simulink model "PID_GM_LastStoer_Kaskadenregler"  (R2021a)
settings: Solver=ode45  StartTime=0.0  StopTime=0.500  RelTol=1e-3  EnableMultiTasking=on
libraries: Regler x3
settings Model: Creator=zimmerma  LastModifiedBy=Manoli
settings SolverCC: AlgebraicLoopSolver=TrustRegion
settings DataIOCC: LimitDataPoints=on  SaveFormat=Array  SignalLoggingSaveFormat=ModelDataLogs  ReturnWorkspaceOutputs=off
settings OptimizationCC: ExpressionDepthLimit=2147483647  InitFltsAndDblsToZero=on  LifeSpan=inf
settings DebuggingCC: SaveWithParameterizedLinksMsg=none  UnderspecifiedInitializationDetection=Classic  MergeDetectMultiDrivingBlocksExec=none  SignalResolutionControl=TryResolveAllWithWarning  MultiTaskDSMMsg=warning  MultiTaskCondExecSysMsg=none  AllowSymbolicDim=off  StateNameClashWarn=warning  SFUnexpectedBacktrackingDiag=warning  SFNoUnconditionalDefaultTransitionDiag=warning  SFExecutionAtInitializationDiag=none  SFMachineParentedDataDiag=warning  ArithmeticOperatorsInVariantConditions=warning
settings HardwareCC: ProdBitPerPointer=32  ProdBitPerSizeT=32  ProdBitPerPtrDiffT=32  ProdLargestAtomicFloat=None  ProdIntDivRoundTo=Undefined  ProdEndianess=Unspecified  ProdWordSize=32  ProdHWDeviceType=32-bit Generic  TargetUnknown=on
settings ModelReferenceCC: PropagateSignalLabelsOutOfModel=off
settings SFSimCC: SimUseLocalCustomCode=off  CustomCodeUndefinedFunction=UseInterfaceOnly
settings RTWCC: RTWUseLocalCustomCode=off
settings CodeAppCC: StateflowObjectComments=on
settings GRTTargetCC: TargetFcnLib=ansi_tfl_tmw.mat  TargetLangStandard=C89/C90 (ANSI)  CombineOutputUpdateFcns=off  GRTInterface=on
settings ConfigComp: CovMetricSettings=dw  CovSaveCumulativeToWorkspaceVar=on  CovSaveSingleToWorkspaceVar=on  CovExternalEMLEnable=off

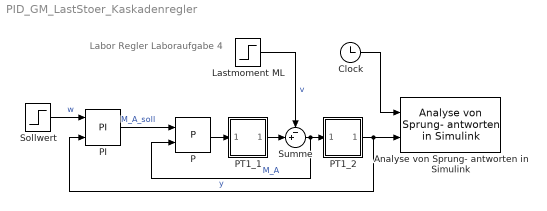
== system PID_GM_LastStoer_Kaskadenregler ==
  note: Labor Regler
      | Laboraufgabe 4
  Analyse von Sprung- antworten in Simulink : Regler/Analyse von Sprung- antworten in Simulink  tol=5
  Clock : Clock
  Lastmoment ML : Step  Time=0.200  SampleTime=0
  P : Regler/P  kp=1
  PI : Regler/PI  kp=10  Tn=100 / 1000
  PT1_1 : Subsystem  mask(PT1){k=4, T1=10 / 1000}
      mask prompts: k "Verstärkung kp"; T1 "Zeitkonstante T1"
      mask help: PT1-Glied kp/(1+s·T1)
      mask Help: PT1 Tiefpaß 1.Ordnung mit Verstärkung kp und Zeitkonstante T1
      mask Display: disp('PT1')
  PT1_2 : Subsystem  mask(PT1){k=1, T1=100 / 1000}
      mask prompts: k "Verstärkung kp"; T1 "Zeitkonstante T1"
      mask help: PT1-Glied kp/(1+s·T1)
      mask Help: PT1 Tiefpaß 1.Ordnung mit Verstärkung kp und Zeitkonstante T1
      mask Display: disp('PT1')
  Sollwert : Step  Time=0  SampleTime=0
  Summe : Sum  Inputs=-+|  InputSameDT=on  SaturateOnIntegerOverflow=on  OutDataTypeStr=Inherit: Same as first input
  wires:
  Sollwert/1 -> PI/1  "w"
  PT1_2/1(Out1) -> Analyse von Sprung- antworten in Simulink/2, PI/2  "y"
  P/1 -> PT1_1/1(In1)
  Summe/1 -> P/2, PT1_2/1(In1)  "M_A"
  PT1_1/1(Out1) -> Summe/2
  Lastmoment ML/1 -> Summe/1  "v"
  Clock/1 -> Analyse von Sprung- antworten in Simulink/1
  PI/1 -> P/1  "M_A_soll"

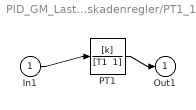
== system PID_GM_LastStoer_Kaskadenregler/PT1_1 ==
  In1 : Inport
  PT1 : TransferFcn  Numerator=[k]  Denominator="[T1  1]"
  Out1 : Outport  VectorParamsAs1DForOutWhenUnconnected=off
  wires:
  In1/1 -> PT1/1
  PT1/1 -> Out1/1

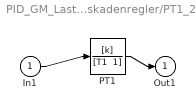
== system PID_GM_LastStoer_Kaskadenregler/PT1_2 ==
  In1 : Inport
  PT1 : TransferFcn  Numerator=[k]  Denominator="[T1  1]"
  Out1 : Outport  VectorParamsAs1DForOutWhenUnconnected=off
  wires:
  PT1/1 -> Out1/1
  In1/1 -> PT1/1
